simulink library "myLibrary"  (R2023b)
settings: Solver=VariableStepAuto  StartTime=0.0  StopTime=10.0  RelTol=1e-3
undefined symbols (not defined in the file): Cac_n1, ctrl1, Da, delta_slk, Discrete, dtha, ee_sli_rtmsupport, FA, gcbh, Ha, Ini, init_DCline, init_IPC, init_line, init_load, init_SG, init_shunt, init_TH, init_trafo, init_user, init_VSC, initMachineBlocks, Ka, Lf, Llkd_pu, Llkq1_pu, magnitude, NET, P, plots_step, q0, Rac_n1, Radd, Rkd_pu, Rkq1_pu, Rload_add, sim_config, sps_rtmsupport, spsSteamTurbineModel, T_DC_NET, T_global, T_IPC, T_load, T_NET, T_SG, T_shunt, T_STATCOM, T_TH, T_trafo, T_user, T_VSC, Ts, tstep, Udiff_a, V1
libraries: spsSeriesRLCBranchLib x120, eeGeneralControl x83, $bdroot x78, spsCurrentMeasurementLib x53, spsParallelRLCBranchLib x39, spsVoltageMeasurementLib x37, spsControlledVoltageSourceLib x30, simulink x29, spsFirstOrderFilterLib x18, spsMeasurementModel x13, spsThreePhaseVIMeasurementLib x5, dspsigops x4
(part 12 of 16)

== system myLibrary/SG_step/Governor-Turbine/Steam Turbine and Governor ==
  wref : Inport
  Pref : Inport  Port=2
  wm : Inport  Port=3
  d_theta : Inport  Port=4
  Model : Subsystem  AncestorBlock=spsSteamTurbineModel/Discrete  DialogController=POWERSYS.PowerSysDialog
      settings: LibrarySourceBlock=spsSteamTurbineModel/Discrete
  dw_5-2 : Outport  VectorParamsAs1DForOutWhenUnconnected=off
  Tr5-2 : Outport  Port=2  VectorParamsAs1DForOutWhenUnconnected=off
  gate : Outport  Port=3  VectorParamsAs1DForOutWhenUnconnected=off
  Pm : Outport  Port=4  VectorParamsAs1DForOutWhenUnconnected=off
  wires:
  wm/1 -> Model/4(wm)
  Model/4(gate) -> gate/1
  Model/3(dw_5-2) -> dw_5-2/1
  d_theta/1 -> Model/3(d_theta)
  Model/2(Tr5-2) -> Tr5-2/1
  Model/1(Pm) -> Pm/1
  wref/1 -> Model/2(wref)
  Pref/1 -> Model/1(Pref)

== system myLibrary/STATCOM/Control/Clarke Anti-Transformation ==
  V_alfa_diff : Inport
  V_beta_dfff : Inport  Port=2
  V_0_diff : Inport  Port=3
  Constant{,2,5,8} (4 alike) : Constant
  Constant1 : Constant  Value=0
  Constant3 : Constant  Value=-1/2
  Constant4 : Constant  Value=-sqrt(3)/2
  Constant6 : Constant  Value=-1/2
  Constant7 : Constant  Value=sqrt(3)/2
  Demux : Demux  Outputs=3
  Display : Display
  Math Function : Math  Operator=transpose  SignedPower=on
  Matrix Concatenate : Concatenate  NumInputs=3  Mode=Multidimensional array  ConcatenateDimension=2
  Mux{,1..3} (4 alike) : Mux  Inputs=3
  Product : Product  Multiplication=Matrix(*)
  Va_diff : Outport  VectorParamsAs1DForOutWhenUnconnected=off
  Vb_diff : Outport  Port=2  VectorParamsAs1DForOutWhenUnconnected=off
  Vc_diff : Outport  Port=3  VectorParamsAs1DForOutWhenUnconnected=off
  wires:
  V_0_diff/1 -> Mux/3  "0"
  V_beta_dfff/1 -> Mux/2  "Vbeta"
  V_alfa_diff/1 -> Mux/1  "Valfa"
  Math Function/1 -> Product/1, Display/1
  Mux/1 -> Product/2
  Demux/3 -> Vc_diff/1  "Vc"
  Demux/2 -> Vb_diff/1  "Vb"
  Demux/1 -> Va_diff/1  "Va"
  Product/1 -> Demux/1
  Mux1/1 -> Matrix Concatenate/1
  Mux3/1 -> Matrix Concatenate/3
  Mux2/1 -> Matrix Concatenate/2
  Matrix Concatenate/1 -> Math Function/1
  Constant8/1 -> Mux3/3
  Constant7/1 -> Mux3/2
  Constant6/1 -> Mux3/1
  Constant5/1 -> Mux2/3
  Constant4/1 -> Mux2/2
  Constant3/1 -> Mux2/1
  Constant2/1 -> Mux1/3
  Constant1/1 -> Mux1/2
  Constant/1 -> Mux1/1

== system myLibrary/STATCOM/Control/Conditional unit delay ==
  In1 : Inport
  Constant4 : Constant  Value=T_VSC.tau_cmd
  Switch : Switch  Criteria=u2 > Threshold  SaturateOnIntegerOverflow=off  InputSameDT=off
  Unit Delay2 : UnitDelay  InitialCondition=initVSC.vdiffq  SampleTime=T_VSC.tau_cmd  HasFrameUpgradeWarning=on
  Out1 : Outport
  wires:
  Switch/1 -> Out1/1
  Unit Delay2/1 -> Switch/1
  In1/1 -> Switch/3, Unit Delay2/1
  Constant4/1 -> Switch/2

== system myLibrary/STATCOM/Control/Conditional zoh ==
  In1 : Inport
  Constant4 : Constant  Value=T_VSC.tau_zoh
  Switch : Switch  Criteria=u2 > Threshold  SaturateOnIntegerOverflow=off  InputSameDT=off
  Zero-Order Hold9 : ZeroOrderHold  SampleTime=T_VSC.tau_zoh
  Out1 : Outport
  wires:
  Switch/1 -> Out1/1
  Constant4/1 -> Switch/2
  Zero-Order Hold9/1 -> Switch/1
  In1/1 -> Switch/3, Zero-Order Hold9/1

== system myLibrary/STATCOM/Control/Current Control ==
  Iq* : Inport
  Iq : Inport  Port=2
  Id* : Inport  Port=3
  Id : Inport  Port=4
  uq : Inport  Port=5
  ud : Inport  Port=6
  Constant : Constant  Value=T_VSC.wb
  Id1 : InportShadow  Port=4
  Integrator : Integrator  InitialCondition=initVSC.PI_idiffq
  Integrator1 : Integrator  InitialCondition=initVSC.PI_idiffd
  Iq1 : InportShadow  Port=2
  Ki : Gain  Gain=T_VSC.ki_s
  Ki1 : Gain  Gain=T_VSC.ki_s
  Kp : Gain  Gain=T_VSC.kp_s
  Kp1 : Gain  Gain=T_VSC.kp_s
  Lc : Gain  Gain=T_VSC.Lc
  Product : Product
  Product1 : Product
  Scope : Scope  NumInputPorts=2
  Sum : Sum  Inputs=|+-
  Sum1 : Sum  Inputs=|+-
  Sum2 : Sum  Inputs=+++
  Sum3 : Sum  Inputs=-++
  Sum4 : Sum
  Sum5 : Sum
  V_q_s : Outport  VectorParamsAs1DForOutWhenUnconnected=off
  V_d_s : Outport  Port=2  VectorParamsAs1DForOutWhenUnconnected=off
  wires:
  Id*/1 -> Sum1/1, Scope/1
  Integrator/1 -> Sum4/1
  Id1/1 -> Product1/2
  Iq1/1 -> Product/1
  Product1/1 -> Sum2/2
  Product/1 -> Sum3/1
  Sum3/1 -> V_d_s/1
  uq/1 -> Sum2/3
  Sum4/1 -> Sum2/1
  ud/1 -> Sum3/3
  Constant/1 -> Lc/1
  Iq*/1 -> Sum/1
  Iq/1 -> Sum/2
  Id/1 -> Sum1/2, Scope/2
  Lc/1 -> Product1/1, Product/2
  Sum/1 -> Ki/1, Kp/1
  Ki/1 -> Integrator/1
  Kp/1 -> Sum4/2
  Sum1/1 -> Kp1/1, Ki1/1  "Error"
  Ki1/1 -> Integrator1/1
  Integrator1/1 -> Sum5/1
  Kp1/1 -> Sum5/2
  Sum5/1 -> Sum3/2
  Sum2/1 -> V_q_s/1

== system myLibrary/STATCOM/Control/DC voltage control ==
  Vdc : Inport
  Constant : Constant
  Integrator : Integrator  InitialCondition=-initVSC.idiffq
  Ki : Gain  Gain=T_VSC.kiVdc
  Kp : Gain  Gain=T_VSC.kpVdc
  Kp1 : Gain  Gain=-1
  Scope : Scope  NumInputPorts=2
  Scope1 : Scope
  Sum1 : Sum  Inputs=|+-
  Sum4 : Sum
  iq : Outport
  wires:
  Constant/1 -> Scope/1, Sum1/1
  Sum1/1 -> Kp/1, Ki/1
  Ki/1 -> Integrator/1
  Sum4/1 -> Kp1/1
  Vdc/1 -> Scope/2, Sum1/2
  Kp1/1 -> Scope1/1, iq/1
  Integrator/1 -> Sum4/1
  Kp/1 -> Sum4/2

== system myLibrary/STATCOM/Control/Is ==
  Ias : Inport
  Ibs : Inport  Port=2
  Ics : Inport  Port=3
  Angle : Inport  Port=4
  Demux1 : Demux  Outputs=3
  Matriu T : Subsystem
  Mux : Mux  Inputs=3
  Product : Product  Multiplication=Matrix(*)
  Terminator : Terminator
  I_q_s : Outport  VectorParamsAs1DForOutWhenUnconnected=off
  I_d_s : Outport  Port=2  VectorParamsAs1DForOutWhenUnconnected=off
  wires:
  Ics/1 -> Mux/3
  Ibs/1 -> Mux/2
  Ias/1 -> Mux/1
  Mux/1 -> Product/2
  Angle/1 -> Matriu T/1(u)
  Demux1/3 -> Terminator/1
  Demux1/2 -> I_d_s/1
  Demux1/1 -> I_q_s/1
  Matriu T/1(Out1) -> Product/1
  Product/1 -> Demux1/1

== system myLibrary/STATCOM/Control/Is1 ==
  Ias : Inport
  Ibs : Inport  Port=2
  Ics : Inport  Port=3
  Angle : Inport  Port=4
  Demux1 : Demux  Outputs=3
  Matriu T : Subsystem
  Mux : Mux  Inputs=3
  Product : Product  Multiplication=Matrix(*)
  I_q_s : Outport  VectorParamsAs1DForOutWhenUnconnected=off
  I_d_s : Outport  Port=2  VectorParamsAs1DForOutWhenUnconnected=off
  I_0_s : Outport  Port=3  VectorParamsAs1DForOutWhenUnconnected=off
  wires:
  Product/1 -> Demux1/1
  Matriu T/1(Out1) -> Product/1
  Demux1/1 -> I_q_s/1
  Demux1/2 -> I_d_s/1
  Demux1/3 -> I_0_s/1
  Angle/1 -> Matriu T/1(u)
  Mux/1 -> Product/2
  Ias/1 -> Mux/1
  Ibs/1 -> Mux/2
  Ics/1 -> Mux/3

== system myLibrary/STATCOM/Control/Is3 ==
  Ias : Inport
  Ibs : Inport  Port=2
  Ics : Inport  Port=3
  Angle : Inport  Port=4
  Demux1 : Demux  Outputs=3
  Matriu T : Subsystem
  Mux : Mux  Inputs=3
  Product : Product  Multiplication=Matrix(*)
  I_q_s : Outport  VectorParamsAs1DForOutWhenUnconnected=off
  I_d_s : Outport  Port=2  VectorParamsAs1DForOutWhenUnconnected=off
  I_0_s : Outport  Port=3  VectorParamsAs1DForOutWhenUnconnected=off
  wires:
  Ics/1 -> Mux/3
  Ibs/1 -> Mux/2
  Ias/1 -> Mux/1
  Mux/1 -> Product/2
  Angle/1 -> Matriu T/1(u)
  Demux1/3 -> I_0_s/1
  Demux1/2 -> I_d_s/1
  Demux1/1 -> I_q_s/1
  Matriu T/1(Out1) -> Product/1
  Product/1 -> Demux1/1

== system myLibrary/STATCOM/Control/Is4 ==
  Ias : Inport
  Ibs : Inport  Port=2
  Ics : Inport  Port=3
  Angle : Inport  Port=4
  Demux1 : Demux  Outputs=3
  Matriu T : Subsystem
  Mux : Mux  Inputs=3
  Product : Product  Multiplication=Matrix(*)
  I_q_s : Outport  VectorParamsAs1DForOutWhenUnconnected=off
  I_d_s : Outport  Port=2  VectorParamsAs1DForOutWhenUnconnected=off
  I_0_s : Outport  Port=3  VectorParamsAs1DForOutWhenUnconnected=off
  wires:
  Product/1 -> Demux1/1
  Matriu T/1(Out1) -> Product/1
  Demux1/1 -> I_q_s/1
  Demux1/2 -> I_d_s/1
  Demux1/3 -> I_0_s/1
  Angle/1 -> Matriu T/1(u)
  Mux/1 -> Product/2
  Ias/1 -> Mux/1
  Ibs/1 -> Mux/2
  Ics/1 -> Mux/3

== system myLibrary/STATCOM/Control/Is5 ==
  Ias : Inport
  Ibs : Inport  Port=2
  Ics : Inport  Port=3
  Angle : Inport  Port=4
  Demux1 : Demux  Outputs=3
  Matriu T : Subsystem
  Mux : Mux  Inputs=3
  Product : Product  Multiplication=Matrix(*)
  I_q_s : Outport  VectorParamsAs1DForOutWhenUnconnected=off
  I_d_s : Outport  Port=2  VectorParamsAs1DForOutWhenUnconnected=off
  I_0_s : Outport  Port=3  VectorParamsAs1DForOutWhenUnconnected=off
  wires:
  Ics/1 -> Mux/3
  Ibs/1 -> Mux/2
  Ias/1 -> Mux/1
  Mux/1 -> Product/2
  Angle/1 -> Matriu T/1(u)
  Demux1/3 -> I_0_s/1
  Demux1/2 -> I_d_s/1
  Demux1/1 -> I_q_s/1
  Matriu T/1(Out1) -> Product/1
  Product/1 -> Demux1/1

== system myLibrary/STATCOM/Control/Is7 ==
  Ias : Inport
  Ibs : Inport  Port=2
  Ics : Inport  Port=3
  Angle : Inport  Port=4
  Demux1 : Demux  Outputs=3
  Matriu T : Subsystem
  Mux : Mux  Inputs=3
  Product : Product  Multiplication=Matrix(*)
  I_q_s : Outport  VectorParamsAs1DForOutWhenUnconnected=off
  I_d_s : Outport  Port=2  VectorParamsAs1DForOutWhenUnconnected=off
  I_0_s : Outport  Port=3  VectorParamsAs1DForOutWhenUnconnected=off
  wires:
  Product/1 -> Demux1/1
  Matriu T/1(Out1) -> Product/1
  Demux1/1 -> I_q_s/1
  Demux1/2 -> I_d_s/1
  Demux1/3 -> I_0_s/1
  Angle/1 -> Matriu T/1(u)
  Mux/1 -> Product/2
  Ias/1 -> Mux/1
  Ibs/1 -> Mux/2
  Ics/1 -> Mux/3

== system myLibrary/STATCOM/Control/PLL ==
  note: PLL
  U : Inport
  Ud : Inport  Port=2
  Constant : Constant  Value=0
  Constant1 : Constant
  Demux : Demux  Outputs=3
  Integrator : Integrator  InitialCondition=initVSC.thetaPLL_init
  Integrator1 : Integrator
  Ki : Gain  Gain=T_VSC.ki_pll
  Kp : Gain  Gain=T_VSC.kp_pll
  Scope1 : Scope
  Scope4 : Scope  NumInputPorts=2
  Sum : Sum  Inputs=|+-
  Sum1 : Sum  Inputs=|++
  Sum2 : Sum  Inputs=|++
  Terminator : Terminator
  Tpark : Subsystem
  wb : Gain  Gain=T_VSC.wb
  Angle : Outport
  Vzq : Outport  Port=2
  Vzd : Outport  Port=3
  w : Outport  Port=4
  wires:
  Ud/1 -> Sum/2, Scope4/2
  Tpark/1(Vq) -> Vzq/1
  U/1 -> Demux/1
  Demux/2 -> Tpark/2(Vb)
  Demux/3 -> Tpark/3(Vc)
  Demux/1 -> Tpark/1(Va)
  Constant/1 -> Sum/1, Scope4/1
  Sum/1 -> Ki/1, Kp/1
  Ki/1 -> Integrator1/1
  Kp/1 -> Sum1/1
  Integrator1/1 -> Sum1/2
  Integrator/1 -> Tpark/4(u), Angle/1
  Tpark/3(0) -> Terminator/1
  Sum1/1 -> Sum2/1
  Constant1/1 -> Sum2/2
  Tpark/2(Vd) -> Vzd/1
  Sum2/1 -> wb/1, Scope1/1
  wb/1 -> w/1, Integrator/1

== system myLibrary/STATCOM/Control/POD ==
  Uq : Inport
  Ud : Inport  Port=2
  iq : Inport  Port=3
  id : Inport  Port=4
  Gain : Gain  Gain=3/2
  LPF : TransferFcn  Denominator=[T_VSC.TLPF 1]
  LeadLag : TransferFcn  Numerator=[T_VSC.T1 1]  Denominator=[T_VSC.T2 1]
  Product : Product
  Product1 : Product
  Sum : Sum
  WashOut : TransferFcn  Numerator=[T_VSC.T 0]  Denominator=[T_VSC.T 1]
  Id_ref : Outport
  wires:
  Uq/1 -> Product/1
  iq/1 -> Product/2
  Ud/1 -> Product1/1
  id/1 -> Product1/2
  Product/1 -> Sum/1
  Product1/1 -> Sum/2
  Sum/1 -> Gain/1
  WashOut/1 -> LeadLag/1
  LeadLag/1 -> Id_ref/1
  LPF/1 -> WashOut/1
  Gain/1 -> LPF/1

== system myLibrary/STATCOM/Control/Rotació ==
  V_q_diff : Inport
  V_d_diff : Inport  Port=2
  V_0_diff : Inport  Port=3
  Angle : Inport  Port=4
  Constant{2,5..7} (4 alike) : Constant  Value=0
  Constant8 : Constant
  Demux : Demux  Outputs=3
  Display : Display
  Gain1 : Gain  Gain=-1
  Matrix Concatenate : Concatenate  NumInputs=3  Mode=Multidimensional array  ConcatenateDimension=2
  Mux{,1..3} (4 alike) : Mux  Inputs=3
  Product : Product  Multiplication=Matrix(*)
  Trigonometric Function : Trigonometry  Operator=cos
  Trigonometric Function1 : Trigonometry
  Trigonometric Function2 : Trigonometry
  Trigonometric Function3 : Trigonometry  Operator=cos
  V_alfa_diff : Outport  VectorParamsAs1DForOutWhenUnconnected=off
  V_beta_diff : Outport  Port=2  VectorParamsAs1DForOutWhenUnconnected=off
  V_0 : Outport  Port=3  VectorParamsAs1DForOutWhenUnconnected=off
  wires:
  Angle/1 -> Trigonometric Function1/1, Trigonometric Function2/1, Trigonometric Function3/1, Trigonometric Function/1
  Trigonometric Function2/1 -> Mux2/1
  Gain1/1 -> Mux1/2
  Trigonometric Function/1 -> Mux1/1
  V_0_diff/1 -> Mux/3
  V_d_diff/1 -> Mux/2
  V_q_diff/1 -> Mux/1
  Matrix Concatenate/1 -> Product/1, Display/1
  Mux/1 -> Product/2
  Demux/3 -> V_0/1
  Demux/2 -> V_beta_diff/1
  Demux/1 -> V_alfa_diff/1
  Product/1 -> Demux/1
  Mux1/1 -> Matrix Concatenate/1
  Mux3/1 -> Matrix Concatenate/3
  Mux2/1 -> Matrix Concatenate/2
  Constant8/1 -> Mux3/3
  Constant7/1 -> Mux3/2
  Constant6/1 -> Mux3/1
  Constant5/1 -> Mux2/3
  Trigonometric Function3/1 -> Mux2/2
  Constant2/1 -> Mux1/3
  Trigonometric Function1/1 -> Gain1/1

== system myLibrary/STATCOM/Control/Subsystem ==
  Uq : Inport
  Ud : Inport  Port=2
  iq : Inport  Port=3
  id : Inport  Port=4
  Gain2 : Gain  Gain=3/2
  Product : Product
  Product1 : Product
  Sum8 : Sum
  Pac : Outport
  wires:
  Uq/1 -> Product/1
  Product/1 -> Sum8/1
  iq/1 -> Product/2
  id/1 -> Product1/2
  Gain2/1 -> Pac/1
  Ud/1 -> Product1/1
  Product1/1 -> Sum8/2
  Sum8/1 -> Gain2/1

== system myLibrary/WT/Control/Clarke Anti-Transformation ==
  V_alfa_diff : Inport
  V_beta_dfff : Inport  Port=2
  V_0_diff : Inport  Port=3
  Constant{,2,5,8} (4 alike) : Constant
  Constant1 : Constant  Value=0
  Constant3 : Constant  Value=-1/2
  Constant4 : Constant  Value=-sqrt(3)/2
  Constant6 : Constant  Value=-1/2
  Constant7 : Constant  Value=sqrt(3)/2
  Demux : Demux  Outputs=3
  Display : Display
  Math Function : Math  Operator=transpose  SignedPower=on
  Matrix Concatenate : Concatenate  NumInputs=3  Mode=Multidimensional array  ConcatenateDimension=2
  Mux{,1..3} (4 alike) : Mux  Inputs=3
  Product : Product  Multiplication=Matrix(*)
  Va_diff : Outport  VectorParamsAs1DForOutWhenUnconnected=off
  Vb_diff : Outport  Port=2  VectorParamsAs1DForOutWhenUnconnected=off
  Vc_diff : Outport  Port=3  VectorParamsAs1DForOutWhenUnconnected=off
  wires:
  V_0_diff/1 -> Mux/3  "0"
  V_beta_dfff/1 -> Mux/2  "Vbeta"
  V_alfa_diff/1 -> Mux/1  "Valfa"
  Math Function/1 -> Product/1, Display/1
  Mux/1 -> Product/2
  Demux/3 -> Vc_diff/1  "Vc"
  Demux/2 -> Vb_diff/1  "Vb"
  Demux/1 -> Va_diff/1  "Va"
  Product/1 -> Demux/1
  Mux1/1 -> Matrix Concatenate/1
  Mux3/1 -> Matrix Concatenate/3
  Mux2/1 -> Matrix Concatenate/2
  Matrix Concatenate/1 -> Math Function/1
  Constant8/1 -> Mux3/3
  Constant7/1 -> Mux3/2
  Constant6/1 -> Mux3/1
  Constant5/1 -> Mux2/3
  Constant4/1 -> Mux2/2
  Constant3/1 -> Mux2/1
  Constant2/1 -> Mux1/3
  Constant1/1 -> Mux1/2
  Constant/1 -> Mux1/1

== system myLibrary/WT/Control/Current Control ==
  Iq* : Inport
  Iq : Inport  Port=2
  Id* : Inport  Port=3
  Id : Inport  Port=4
  uq : Inport  Port=5
  ud : Inport  Port=6
  igq : Inport  Port=7
  igd : Inport  Port=8
  Constant : Constant  Value=T_VSC.wb
  Gain1 : Gain  Gain=T_VSC.cc_damp
  Gain2 : Gain  Gain=T_VSC.cc_damp
  Id1 : InportShadow  Port=4
  Id2 : InportShadow  Port=4
  Integrator : Integrator  InitialCondition=initVSC.PI_idiffq
  Integrator1 : Integrator  InitialCondition=initVSC.PI_idiffd
  Iq1 : InportShadow  Port=2
  Iq2 : InportShadow  Port=2
  Ki : Gain  Gain=T_VSC.ki_s
  Ki1 : Gain  Gain=T_VSC.ki_s
  Kp : Gain  Gain=T_VSC.kp_s
  Kp1 : Gain  Gain=T_VSC.kp_s
  Lc : Gain  Gain=T_VSC.Lc
  Lc1 : Gain  Gain=T_VSC.Rc*T_VSC.Lc*T_VSC.wb
  Lc2 : Gain  Gain=T_VSC.Rc*T_VSC.Lc*T_VSC.wb
  Product : Product
  Product1 : Product
  Scope : Scope  NumInputPorts=2
  Scope{1..4} (4 alike) : Scope
  Sum{,1,8..9} (4 alike) : Sum  Inputs=|+-
  Sum2 : Sum  Inputs=+++++
  Sum3 : Sum  Inputs=+-+++
  Sum4 : Sum
  Sum5 : Sum
  V_q_s : Outport  VectorParamsAs1DForOutWhenUnconnected=off
  V_d_s : Outport  Port=2  VectorParamsAs1DForOutWhenUnconnected=off
  wires:
  Id*/1 -> Sum1/1, Scope/1
  Integrator/1 -> Scope3/1, Sum4/1
  Id1/1 -> Lc1/1, Product1/2
  Iq1/1 -> Lc2/1, Product/1
  Sum3/1 -> Scope2/1, V_d_s/1
  Sum4/1 -> Sum2/2
  Constant/1 -> Lc/1
  Iq*/1 -> Sum/1
  Iq/1 -> Sum/2
  Id/1 -> Sum1/2, Scope/2
  Lc/1 -> Product1/1, Product/2
  Sum/1 -> Ki/1, Kp/1
  Ki/1 -> Integrator/1
  Kp/1 -> Sum4/2
  Sum1/1 -> Kp1/1, Ki1/1  "Error"
  Ki1/1 -> Integrator1/1
  Integrator1/1 -> Scope4/1, Sum5/1
  Kp1/1 -> Sum5/2
  Sum2/1 -> Scope1/1, V_q_s/1
  ud/1 -> Sum3/1
  igq/1 -> Sum8/1
  Gain1/1 -> Sum2/1
  Iq2/1 -> Sum8/2
  Sum8/1 -> Gain1/1
  igd/1 -> Sum9/1
  Id2/1 -> Sum9/2
  Sum9/1 -> Gain2/1
  uq/1 -> Sum2/5
  Gain2/1 -> Sum3/5
  Sum5/1 -> Sum3/4
  Lc2/1 -> Sum2/3
  Product1/1 -> Sum2/4
  Product/1 -> Sum3/2
  Lc1/1 -> Sum3/3

== system myLibrary/WT/Control/DC voltage control ==
  Vdc : Inport
  Constant : Constant  Value=2*sqrt(3/2)
  Integrator : Integrator  InitialCondition=-initVSC.idiffqc_p
  Ki : Gain  Gain=T_VSC.kiVdc
  Kp : Gain  Gain=T_VSC.kpVdc
  Kp1 : Gain  Gain=-1
  Scope : Scope  NumInputPorts=2
  Scope1 : Scope
  Scope2 : Scope
  Sum1 : Sum  Inputs=|+-
  Sum4 : Sum
  iq : Outport
  wires:
  Constant/1 -> Scope/1, Sum1/1
  Sum1/1 -> Kp/1, Ki/1
  Ki/1 -> Integrator/1
  Sum4/1 -> Kp1/1
  Vdc/1 -> Scope/2, Sum1/2
  Kp1/1 -> Scope1/1, iq/1
  Integrator/1 -> Scope2/1, Sum4/1
  Kp/1 -> Sum4/2

== system myLibrary/WT/Control/Is ==
  Ias : Inport
  Ibs : Inport  Port=2
  Ics : Inport  Port=3
  Angle : Inport  Port=4
  Demux1 : Demux  Outputs=3
  Matriu T : Subsystem
  Mux : Mux  Inputs=3
  Product : Product  Multiplication=Matrix(*)
  Terminator : Terminator
  I_q_s : Outport  VectorParamsAs1DForOutWhenUnconnected=off
  I_d_s : Outport  Port=2  VectorParamsAs1DForOutWhenUnconnected=off
  wires:
  Ics/1 -> Mux/3
  Ibs/1 -> Mux/2
  Ias/1 -> Mux/1
  Mux/1 -> Product/2
  Angle/1 -> Matriu T/1(u)
  Demux1/3 -> Terminator/1
  Demux1/2 -> I_d_s/1
  Demux1/1 -> I_q_s/1
  Matriu T/1(Out1) -> Product/1
  Product/1 -> Demux1/1

== system myLibrary/WT/Control/Is1 ==
  Ias : Inport
  Ibs : Inport  Port=2
  Ics : Inport  Port=3
  Angle : Inport  Port=4
  Demux1 : Demux  Outputs=3
  Matriu T : Subsystem
  Mux : Mux  Inputs=3
  Product : Product  Multiplication=Matrix(*)
  I_q_s : Outport  VectorParamsAs1DForOutWhenUnconnected=off
  I_d_s : Outport  Port=2  VectorParamsAs1DForOutWhenUnconnected=off
  I_0_s : Outport  Port=3  VectorParamsAs1DForOutWhenUnconnected=off
  wires:
  Product/1 -> Demux1/1
  Matriu T/1(Out1) -> Product/1
  Demux1/1 -> I_q_s/1
  Demux1/2 -> I_d_s/1
  Demux1/3 -> I_0_s/1
  Angle/1 -> Matriu T/1(u)
  Mux/1 -> Product/2
  Ias/1 -> Mux/1
  Ibs/1 -> Mux/2
  Ics/1 -> Mux/3

== system myLibrary/WT/Control/Is3 ==
  Ias : Inport
  Ibs : Inport  Port=2
  Ics : Inport  Port=3
  Angle : Inport  Port=4
  Demux1 : Demux  Outputs=3
  Matriu T : Subsystem
  Mux : Mux  Inputs=3
  Product : Product  Multiplication=Matrix(*)
  I_q_s : Outport  VectorParamsAs1DForOutWhenUnconnected=off
  I_d_s : Outport  Port=2  VectorParamsAs1DForOutWhenUnconnected=off
  I_0_s : Outport  Port=3  VectorParamsAs1DForOutWhenUnconnected=off
  wires:
  Ics/1 -> Mux/3
  Ibs/1 -> Mux/2
  Ias/1 -> Mux/1
  Mux/1 -> Product/2
  Angle/1 -> Matriu T/1(u)
  Demux1/3 -> I_0_s/1
  Demux1/2 -> I_d_s/1
  Demux1/1 -> I_q_s/1
  Matriu T/1(Out1) -> Product/1
  Product/1 -> Demux1/1

== system myLibrary/WT/Control/Is4 ==
  Ias : Inport
  Ibs : Inport  Port=2
  Ics : Inport  Port=3
  Angle : Inport  Port=4
  Demux1 : Demux  Outputs=3
  Matriu T : Subsystem
  Mux : Mux  Inputs=3
  Product : Product  Multiplication=Matrix(*)
  I_q_s : Outport  VectorParamsAs1DForOutWhenUnconnected=off
  I_d_s : Outport  Port=2  VectorParamsAs1DForOutWhenUnconnected=off
  I_0_s : Outport  Port=3  VectorParamsAs1DForOutWhenUnconnected=off
  wires:
  Product/1 -> Demux1/1
  Matriu T/1(Out1) -> Product/1
  Demux1/1 -> I_q_s/1
  Demux1/2 -> I_d_s/1
  Demux1/3 -> I_0_s/1
  Angle/1 -> Matriu T/1(u)
  Mux/1 -> Product/2
  Ias/1 -> Mux/1
  Ibs/1 -> Mux/2
  Ics/1 -> Mux/3

== system myLibrary/WT/Control/Is5 ==
  Ias : Inport
  Ibs : Inport  Port=2
  Ics : Inport  Port=3
  Angle : Inport  Port=4
  Demux1 : Demux  Outputs=3
  Matriu T : Subsystem
  Mux : Mux  Inputs=3
  Product : Product  Multiplication=Matrix(*)
  I_q_s : Outport  VectorParamsAs1DForOutWhenUnconnected=off
  I_d_s : Outport  Port=2  VectorParamsAs1DForOutWhenUnconnected=off
  I_0_s : Outport  Port=3  VectorParamsAs1DForOutWhenUnconnected=off
  wires:
  Ics/1 -> Mux/3
  Ibs/1 -> Mux/2
  Ias/1 -> Mux/1
  Mux/1 -> Product/2
  Angle/1 -> Matriu T/1(u)
  Demux1/3 -> I_0_s/1
  Demux1/2 -> I_d_s/1
  Demux1/1 -> I_q_s/1
  Matriu T/1(Out1) -> Product/1
  Product/1 -> Demux1/1

== system myLibrary/WT/Control/Is7 ==
  Ias : Inport
  Ibs : Inport  Port=2
  Ics : Inport  Port=3
  Angle : Inport  Port=4
  Demux1 : Demux  Outputs=3
  Matriu T : Subsystem
  Mux : Mux  Inputs=3
  Product : Product  Multiplication=Matrix(*)
  I_q_s : Outport  VectorParamsAs1DForOutWhenUnconnected=off
  I_d_s : Outport  Port=2  VectorParamsAs1DForOutWhenUnconnected=off
  I_0_s : Outport  Port=3  VectorParamsAs1DForOutWhenUnconnected=off
  wires:
  Product/1 -> Demux1/1
  Matriu T/1(Out1) -> Product/1
  Demux1/1 -> I_q_s/1
  Demux1/2 -> I_d_s/1
  Demux1/3 -> I_0_s/1
  Angle/1 -> Matriu T/1(u)
  Mux/1 -> Product/2
  Ias/1 -> Mux/1
  Ibs/1 -> Mux/2
  Ics/1 -> Mux/3

== system myLibrary/WT/Control/Is8 ==
  Ias : Inport
  Ibs : Inport  Port=2
  Ics : Inport  Port=3
  Angle : Inport  Port=4
  Demux1 : Demux  Outputs=3
  Matriu T : Subsystem
  Mux : Mux  Inputs=3
  Product : Product  Multiplication=Matrix(*)
  I_q_s : Outport  VectorParamsAs1DForOutWhenUnconnected=off
  I_d_s : Outport  Port=2  VectorParamsAs1DForOutWhenUnconnected=off
  I_0_s : Outport  Port=3  VectorParamsAs1DForOutWhenUnconnected=off
  wires:
  Ics/1 -> Mux/3
  Ibs/1 -> Mux/2
  Ias/1 -> Mux/1
  Mux/1 -> Product/2
  Angle/1 -> Matriu T/1(u)
  Demux1/3 -> I_0_s/1
  Demux1/2 -> I_d_s/1
  Demux1/1 -> I_q_s/1
  Matriu T/1(Out1) -> Product/1
  Product/1 -> Demux1/1

== system myLibrary/WT/Control/Low-Pass Filter (Discrete or Continuous)2 ==
  u : Inport
  1/T : Product  Inputs=/*
  Enable/disable time constant : Subsystem
  Initialization : Subsystem  Variant=on  VariantControlMode=label  LabelModeActiveChoice=Init_param
  Integrator (Discrete or Continuous) : eeGeneralControl/Integrator (Discrete or Continuous)  LabelModeActiveChoice=Discrete  ExternalReset=level  LimitType=Anti-windup  B=B  A=A  Ts=Ts
      settings: LibrarySourceBlock=|
      | ee_sl_lib/General Control/Low-Pass Filter
      | (Discrete or Continuous)/Integrator
      | (Discrete or Continuous)
  K : Gain  Gain=K
  Sum1 : Sum  Inputs=-+|
  y : Outport  VectorParamsAs1DForOutWhenUnconnected=off
  wires:
  Initialization/1(x0) -> Integrator (Discrete or Continuous)/3
  u/1 -> K/1
  Enable/disable time constant/2(reset) -> Integrator (Discrete or Continuous)/2
  Integrator (Discrete or Continuous)/1 -> y/1, Enable/disable time constant/1(x), Sum1/1
  Enable/disable time constant/1(max(T,Ts)) -> 1/T/1
  1/T/1 -> Integrator (Discrete or Continuous)/1
  Sum1/1 -> 1/T/2
  K/1 -> Sum1/2, Initialization/1(u)

== system myLibrary/WT/Control/Low-Pass Filter (Discrete or Continuous)3 ==
  u : Inport
  1/T : Product  Inputs=/*
  Enable/disable time constant : Subsystem
  Initialization : Subsystem  Variant=on  VariantControlMode=label  LabelModeActiveChoice=Init_param
  Integrator (Discrete or Continuous) : eeGeneralControl/Integrator (Discrete or Continuous)  LabelModeActiveChoice=Discrete  ExternalReset=level  LimitType=Anti-windup  B=B  A=A  Ts=Ts
      settings: LibrarySourceBlock=|
      | ee_sl_lib/General Control/Low-Pass Filter
      | (Discrete or Continuous)/Integrator
      | (Discrete or Continuous)
  K : Gain  Gain=K
  Sum1 : Sum  Inputs=-+|
  y : Outport  VectorParamsAs1DForOutWhenUnconnected=off
  wires:
  Initialization/1(x0) -> Integrator (Discrete or Continuous)/3
  u/1 -> K/1
  Enable/disable time constant/2(reset) -> Integrator (Discrete or Continuous)/2
  Integrator (Discrete or Continuous)/1 -> y/1, Enable/disable time constant/1(x), Sum1/1
  Enable/disable time constant/1(max(T,Ts)) -> 1/T/1
  1/T/1 -> Integrator (Discrete or Continuous)/1
  Sum1/1 -> 1/T/2
  K/1 -> Sum1/2, Initialization/1(u)

== system myLibrary/WT/Control/Low-Pass Filter (Discrete or Continuous)4 ==
  u : Inport
  1/T : Product  Inputs=/*
  Enable/disable time constant : Subsystem
  Initialization : Subsystem  Variant=on  VariantControlMode=label  LabelModeActiveChoice=Init_param
  Integrator (Discrete or Continuous) : eeGeneralControl/Integrator (Discrete or Continuous)  LabelModeActiveChoice=Discrete  ExternalReset=level  LimitType=Anti-windup  B=B  A=A  Ts=Ts
      settings: LibrarySourceBlock=|
      | eeGeneralControl/Low-Pass Filter
      | (Discrete or Continuous)/Integrator
      | (Discrete or Continuous)
  K : Gain  Gain=K
  Sum1 : Sum  Inputs=-+|
  y : Outport  VectorParamsAs1DForOutWhenUnconnected=off
  wires:
  Initialization/1(x0) -> Integrator (Discrete or Continuous)/3
  u/1 -> K/1
  Enable/disable time constant/2(reset) -> Integrator (Discrete or Continuous)/2
  Integrator (Discrete or Continuous)/1 -> y/1, Enable/disable time constant/1(x), Sum1/1
  Enable/disable time constant/1(max(T,Ts)) -> 1/T/1
  1/T/1 -> Integrator (Discrete or Continuous)/1
  Sum1/1 -> 1/T/2
  K/1 -> Sum1/2, Initialization/1(u)

== system myLibrary/WT/Control/Low-Pass Filter (Discrete or Continuous)5 ==
  u : Inport
  1/T : Product  Inputs=/*
  Enable/disable time constant : Subsystem
  Initialization : Subsystem  Variant=on  VariantControlMode=label  LabelModeActiveChoice=Init_param
  Integrator (Discrete or Continuous) : eeGeneralControl/Integrator (Discrete or Continuous)  LabelModeActiveChoice=Discrete  ExternalReset=level  LimitType=Anti-windup  B=B  A=A  Ts=Ts
      settings: LibrarySourceBlock=|
      | ee_sl_lib/General Control/Low-Pass Filter
      | (Discrete or Continuous)/Integrator
      | (Discrete or Continuous)
  K : Gain  Gain=K
  Sum1 : Sum  Inputs=-+|
  y : Outport  VectorParamsAs1DForOutWhenUnconnected=off
  wires:
  K/1 -> Initialization/1(u), Sum1/2
  Sum1/1 -> 1/T/2
  1/T/1 -> Integrator (Discrete or Continuous)/1
  Enable/disable time constant/1(max(T,Ts)) -> 1/T/1
  Integrator (Discrete or Continuous)/1 -> Sum1/1, Enable/disable time constant/1(x), y/1
  Enable/disable time constant/2(reset) -> Integrator (Discrete or Continuous)/2
  u/1 -> K/1
  Initialization/1(x0) -> Integrator (Discrete or Continuous)/3

== system myLibrary/WT/Control/Low-Pass Filter (Discrete or Continuous)6 ==
  u : Inport
  1/T : Product  Inputs=/*
  Enable/disable time constant : Subsystem
  Initialization : Subsystem  Variant=on  VariantControlMode=label  LabelModeActiveChoice=Init_param
  Integrator (Discrete or Continuous) : eeGeneralControl/Integrator (Discrete or Continuous)  LabelModeActiveChoice=Discrete  ExternalReset=level  LimitType=Anti-windup  B=B  A=A  Ts=Ts
      settings: LibrarySourceBlock=|
      | ee_sl_lib/General Control/Low-Pass Filter
      | (Discrete or Continuous)/Integrator
      | (Discrete or Continuous)
  K : Gain  Gain=K
  Sum1 : Sum  Inputs=-+|
  y : Outport  VectorParamsAs1DForOutWhenUnconnected=off
  wires:
  K/1 -> Initialization/1(u), Sum1/2
  Sum1/1 -> 1/T/2
  1/T/1 -> Integrator (Discrete or Continuous)/1
  Enable/disable time constant/1(max(T,Ts)) -> 1/T/1
  Integrator (Discrete or Continuous)/1 -> Sum1/1, Enable/disable time constant/1(x), y/1
  Enable/disable time constant/2(reset) -> Integrator (Discrete or Continuous)/2
  u/1 -> K/1
  Initialization/1(x0) -> Integrator (Discrete or Continuous)/3

== system myLibrary/WT/Control/Low-Pass Filter (Discrete or Continuous)7 ==
  u : Inport
  1/T : Product  Inputs=/*
  Enable/disable time constant : Subsystem
  Initialization : Subsystem  Variant=on  VariantControlMode=label  LabelModeActiveChoice=Init_param
  Integrator (Discrete or Continuous) : eeGeneralControl/Integrator (Discrete or Continuous)  LabelModeActiveChoice=Discrete  ExternalReset=level  LimitType=Anti-windup  B=B  A=A  Ts=Ts
      settings: LibrarySourceBlock=|
      | ee_sl_lib/General Control/Low-Pass Filter
      | (Discrete or Continuous)/Integrator
      | (Discrete or Continuous)
  K : Gain  Gain=K
  Sum1 : Sum  Inputs=-+|
  y : Outport  VectorParamsAs1DForOutWhenUnconnected=off
  wires:
  Initialization/1(x0) -> Integrator (Discrete or Continuous)/3
  u/1 -> K/1
  Enable/disable time constant/2(reset) -> Integrator (Discrete or Continuous)/2
  Integrator (Discrete or Continuous)/1 -> y/1, Enable/disable time constant/1(x), Sum1/1
  Enable/disable time constant/1(max(T,Ts)) -> 1/T/1
  1/T/1 -> Integrator (Discrete or Continuous)/1
  Sum1/1 -> 1/T/2
  K/1 -> Sum1/2, Initialization/1(u)

== system myLibrary/WT/Control/Low-Pass Filter (Discrete or Continuous)8 ==
  u : Inport
  1/T : Product  Inputs=/*
  Enable/disable time constant : Subsystem
  Initialization : Subsystem  Variant=on  VariantControlMode=label  LabelModeActiveChoice=Init_param
  Integrator (Discrete or Continuous) : eeGeneralControl/Integrator (Discrete or Continuous)  LabelModeActiveChoice=Discrete  ExternalReset=level  LimitType=Anti-windup  B=B  A=A  Ts=Ts
      settings: LibrarySourceBlock=|
      | ee_sl_lib/General Control/Low-Pass Filter
      | (Discrete or Continuous)/Integrator
      | (Discrete or Continuous)
  K : Gain  Gain=K
  Sum1 : Sum  Inputs=-+|
  y : Outport  VectorParamsAs1DForOutWhenUnconnected=off
  wires:
  Initialization/1(x0) -> Integrator (Discrete or Continuous)/3
  u/1 -> K/1
  Enable/disable time constant/2(reset) -> Integrator (Discrete or Continuous)/2
  Integrator (Discrete or Continuous)/1 -> y/1, Enable/disable time constant/1(x), Sum1/1
  Enable/disable time constant/1(max(T,Ts)) -> 1/T/1
  1/T/1 -> Integrator (Discrete or Continuous)/1
  Sum1/1 -> 1/T/2
  K/1 -> Sum1/2, Initialization/1(u)

== system myLibrary/WT/Control/Low-Pass Filter (Discrete or Continuous)9 ==
  u : Inport
  1/T : Product  Inputs=/*
  Enable/disable time constant : Subsystem
  Initialization : Subsystem  Variant=on  VariantControlMode=label  LabelModeActiveChoice=Init_param
  Integrator (Discrete or Continuous) : eeGeneralControl/Integrator (Discrete or Continuous)  LabelModeActiveChoice=Discrete  ExternalReset=level  LimitType=Anti-windup  B=B  A=A  Ts=Ts
      settings: LibrarySourceBlock=|
      | ee_sl_lib/General Control/Low-Pass Filter
      | (Discrete or Continuous)/Integrator
      | (Discrete or Continuous)
  K : Gain  Gain=K
  Sum1 : Sum  Inputs=-+|
  y : Outport  VectorParamsAs1DForOutWhenUnconnected=off
  wires:
  K/1 -> Initialization/1(u), Sum1/2
  Sum1/1 -> 1/T/2
  1/T/1 -> Integrator (Discrete or Continuous)/1
  Enable/disable time constant/1(max(T,Ts)) -> 1/T/1
  Integrator (Discrete or Continuous)/1 -> Sum1/1, Enable/disable time constant/1(x), y/1
  Enable/disable time constant/2(reset) -> Integrator (Discrete or Continuous)/2
  u/1 -> K/1
  Initialization/1(x0) -> Integrator (Discrete or Continuous)/3

== system myLibrary/WT/Control/PLL ==
  note: PLL
  U : Inport
  Constant : Constant  Value=0
  Constant1 : Constant
  Demux : Demux  Outputs=3
  Integrator : Integrator  InitialCondition=initVSC.thetaPLL_init_filts
  Integrator1 : Integrator
  Ki : Gain  Gain=T_VSC.ki_pll
  Kp : Gain  Gain=T_VSC.kp_pll
  Low-Pass Filter (Discrete or Continuous)1 : Subsystem  LoadFcn=ee_sli_rtmsupport( 'loadfcn', gcbh );  mask(Low-Pass Filter (Discrete or Continuous)){K=1, T=0, B=inf, A=-inf, init_option=Specify as parameter, x0=initVSC.udc_p, Ts=-1}
      mask prompts: K "physmod:ee:library:comments:control:eeGeneralControl:Gain_MP"; T "physmod:ee:library:comments:control:eeGeneralControl:TimeConstant_MP"; B "physmod:ee:library:comments:control:eeGeneralControl:UpperSaturationLimit_MP"; A "physmod:ee:library:comments:control:eeGeneralControl:LowerSaturationLimit_MP"; init_option "physmod:ee:library:comments:control:eeGeneralControl:Initialization_MP"; x0 "physmod:ee:library:comments:control:eeGeneralControl:InitialState_MP"; Ts "physmod:ee:library:comments:control:eeGeneralControl:SampleTime1ForInherited_MP"
      mask help: physmod:ee:library:comments:control:eeGeneralControl:LowPassFilterDiscreteOrContinuous_MD
      mask init:
      | timeDomain = ee.mask.initializeLowPassFilter(T,B,A,Ts);
      | 
      | ee.mask.callbackPopupInitialization(gcb);
      settings: CopyFcn=ee_sli_rtmsupport( 'copyfcn', gcbh );  DeleteFcn=ee_sli_rtmsupport( 'deletefcn', gcbh );  ModelCloseFcn=ee_sli_rtmsupport( 'modelclosefcn', gcbh );  PostSaveFcn=ee_sli_rtmsupport( 'postsavefcn', gcbh );  PreCopyFcn=ee_sli_rtmsupport( 'precopyfcn', gcbh );  OpenFcn=ee_sli_rtmsupport( 'openfcn', gcbh );  CloseFcn=ee_sli_rtmsupport( 'closefcn', gcbh );  PreDeleteFcn=ee_sli_rtmsupport( 'predeletefcn', gcbh );
      settings: LibrarySourceBlock=|
      | eeGeneralControl/Low-Pass Filter
      | (Discrete or Continuous)
      mask Help: web(nesl_help(gcbh))
      mask TypeOptions init_option: physmod:ee:library:comments:control:eeGeneralControl:InheritedFromBlockInput_PV | physmod:ee:library:comments:control:eeGeneralControl:SpecifyAsParameter_PV
      mask Callback init_option: ee.mask.callbackPopupInitialization(gcb);
      mask TypeOptions Ts:
      | Integrator
      | (Discrete or Continuous)/Ts
      mask DialogControl ParameterGroupVar Prompt: physmod:ee:library:comments:control:eeGeneralControl:tab_Parameters
      mask DialogControl K Prompt: Gain
      mask DialogControl T Prompt: Time constant
      mask DialogControl B Prompt: Upper saturation limit
      mask DialogControl A Prompt: Lower saturation limit
      mask DialogControl init_option Prompt: Initialization
      mask DialogControl x0 Prompt: Initial state
      mask DialogControl Ts Prompt: Sample time (-1 for inherited)
      mask Display: ee.mask.drawLowPassFilter;
  Sum : Sum  Inputs=|+-
  Sum1 : Sum  Inputs=|++
  Sum2 : Sum  Inputs=|++
  Terminator : Terminator
  Tpark : Subsystem
  wb : Gain  Gain=T_VSC.wb
  Angle : Outport
  Vzq : Outport  Port=2
  Vzd : Outport  Port=3
  w : Outport  Port=4
  wires:
  Tpark/1(Vq) -> Vzq/1
  U/1 -> Demux/1
  Demux/2 -> Tpark/2(Vb)
  Demux/3 -> Tpark/3(Vc)
  Demux/1 -> Tpark/1(Va)
  Constant/1 -> Sum/1
  Sum/1 -> Ki/1, Kp/1
  Ki/1 -> Integrator1/1
  Kp/1 -> Sum1/1
  Integrator1/1 -> Sum1/2
  Integrator/1 -> Tpark/4(u), Angle/1
  Tpark/3(0) -> Terminator/1
  Sum1/1 -> Sum2/1
  Constant1/1 -> Sum2/2
  Tpark/2(Vd) -> Low-Pass Filter (Discrete or Continuous)1/1(u), Vzd/1
  Sum2/1 -> wb/1
  wb/1 -> w/1, Integrator/1
  Low-Pass Filter (Discrete or Continuous)1/1(y) -> Sum/2

== system myLibrary/WT/Control/Q control ==
  Q : Inport
  Integrator : Integrator  InitialCondition=initVSC.idiffdc_p
  Ki : Gain  Gain=T_VSC.ki_Q
  Kp : Gain  Gain=T_VSC.kp_Q
  Kp1 : Gain
  Scope : Scope
  Scope1 : Scope
  Sum4 : Sum
  id : Outport
  wires:
  Kp/1 -> Sum4/2
  Integrator/1 -> Scope/1, Sum4/1
  Kp1/1 -> id/1, Scope1/1
  Sum4/1 -> Kp1/1
  Ki/1 -> Integrator/1
  Q/1 -> Kp/1, Ki/1

== system myLibrary/WT/Control/Rotació ==
  V_q_diff : Inport
  V_d_diff : Inport  Port=2
  V_0_diff : Inport  Port=3
  Angle : Inport  Port=4
  Constant{2,5..7} (4 alike) : Constant  Value=0
  Constant8 : Constant
  Demux : Demux  Outputs=3
  Display : Display
  Gain1 : Gain  Gain=-1
  Matrix Concatenate : Concatenate  NumInputs=3  Mode=Multidimensional array  ConcatenateDimension=2
  Mux{,1..3} (4 alike) : Mux  Inputs=3
  Product : Product  Multiplication=Matrix(*)
  Trigonometric Function : Trigonometry  Operator=cos
  Trigonometric Function1 : Trigonometry
  Trigonometric Function2 : Trigonometry
  Trigonometric Function3 : Trigonometry  Operator=cos
  V_alfa_diff : Outport  VectorParamsAs1DForOutWhenUnconnected=off
  V_beta_diff : Outport  Port=2  VectorParamsAs1DForOutWhenUnconnected=off
  V_0 : Outport  Port=3  VectorParamsAs1DForOutWhenUnconnected=off
  wires:
  Angle/1 -> Trigonometric Function1/1, Trigonometric Function2/1, Trigonometric Function3/1, Trigonometric Function/1
  Trigonometric Function2/1 -> Mux2/1
  Gain1/1 -> Mux1/2
  Trigonometric Function/1 -> Mux1/1
  V_0_diff/1 -> Mux/3
  V_d_diff/1 -> Mux/2
  V_q_diff/1 -> Mux/1
  Matrix Concatenate/1 -> Product/1, Display/1
  Mux/1 -> Product/2
  Demux/3 -> V_0/1
  Demux/2 -> V_beta_diff/1
  Demux/1 -> V_alfa_diff/1
  Product/1 -> Demux/1
  Mux1/1 -> Matrix Concatenate/1
  Mux3/1 -> Matrix Concatenate/3
  Mux2/1 -> Matrix Concatenate/2
  Constant8/1 -> Mux3/3
  Constant7/1 -> Mux3/2
  Constant6/1 -> Mux3/1
  Constant5/1 -> Mux2/3
  Trigonometric Function3/1 -> Mux2/2
  Constant2/1 -> Mux1/3
  Trigonometric Function1/1 -> Gain1/1

== system myLibrary/WT/Control/Subsystem ==
  Uq : Inport
  Ud : Inport  Port=2
  iq : Inport  Port=3
  id : Inport  Port=4
  Product : Product
  Product1 : Product
  Sum8 : Sum
  Pac : Outport
  wires:
  Uq/1 -> Product/1
  Product/1 -> Sum8/1
  iq/1 -> Product/2
  id/1 -> Product1/2
  Sum8/1 -> Pac/1
  Ud/1 -> Product1/1
  Product1/1 -> Sum8/2

== system myLibrary/WT/Control/Subsystem1 ==
  Uq : Inport
  Ud : Inport  Port=2
  iq : Inport  Port=3
  id : Inport  Port=4
  Product : Product
  Product1 : Product
  Sum8 : Sum  Inputs=+-
  Qac : Outport
  wires:
  Product1/1 -> Sum8/2
  Ud/1 -> Product1/1
  Sum8/1 -> Qac/1
  Product/1 -> Sum8/1
  Uq/1 -> Product/1
  id/1 -> Product/2
  iq/1 -> Product1/2

== system myLibrary/WT/Electrical/Power7 ==
  Vabc : Inport  PortDimensions=3
  Iabc : Inport  Port=2  PortDimensions=3
  Demux : Demux  Outputs=3
      settings: DisplayOption=none
  Mux : Mux  Inputs=3
  Product1 : Product  InputSameDT=on  SaturateOnIntegerOverflow=on  OutDataTypeStr=Inherit: Same as first input
  Product3 : Product  InputSameDT=on  SaturateOnIntegerOverflow=on  OutDataTypeStr=Inherit: Same as first input
  Sum : Sum  Inputs=+-  InputSameDT=on  SaturateOnIntegerOverflow=on  OutDataTypeStr=Inherit: Same as first input
  Sum1 : Sum  Inputs=1  InputSameDT=on  SaturateOnIntegerOverflow=on  OutDataTypeStr=Inherit: Same as first input
  Sum4 : Sum  Inputs=1  InputSameDT=on  SaturateOnIntegerOverflow=on  OutDataTypeStr=Inherit: Same as first input
  Sum5 : Sum  Inputs=+-  InputSameDT=on  SaturateOnIntegerOverflow=on  OutDataTypeStr=Inherit: Same as first input
  Sum6 : Sum  Inputs=+-  InputSameDT=on  SaturateOnIntegerOverflow=on  OutDataTypeStr=Inherit: Same as first input
  pu->V : Gain  Gain=1/sqrt(3)  SaturateOnIntegerOverflow=on  OutDataTypeStr=Inherit: Same as input  ParamDataTypeStr=Inherit: Same as input
  P : Outport  VectorParamsAs1DForOutWhenUnconnected=off
  Q : Outport  Port=2  VectorParamsAs1DForOutWhenUnconnected=off
  wires:
  pu->V/1 -> Q/1
  Sum4/1 -> P/1
  Sum1/1 -> pu->V/1
  Product3/1 -> Sum1/1
  Product1/1 -> Sum4/1
  Vabc/1 -> Product1/1, Demux/1
  Iabc/1 -> Product1/2, Product3/2
  Demux/1 -> Sum/1, Sum6/2
  Demux/2 -> Sum/2, Sum5/1
  Demux/3 -> Sum5/2, Sum6/1
  Sum/1 -> Mux/3
  Sum5/1 -> Mux/1
  Sum6/1 -> Mux/2
  Mux/1 -> Product3/1

== system myLibrary/WT/Electrical/Voltage Measurement1 ==
  Model : spsMeasurementModel/Complex  SystemSampleTime=-1  VariantActivationTime=update diagram  AllowFlexibleInterface=on  Latency=0  AutoFrameSizeCalculation=off
      settings: LibrarySourceBlock=sps_lib/Sensors and Measurements/Voltage Measurement/Model
  VoltageMeasurement : PMComponent  PhysicalDomain=powersysdomain  LeftPortType=p1  RightPortType=p1  LConnTagsString=+  RConnTagsString=-  mask(InnerPowersysBlock){}
      mask Display: disp('SPS internal use\nDo not delete')
  do not delete this gain : Gain
  + : PMIOPort  Side=Left
  - : PMIOPort  Port=2  Side=Left
  v : Outport  InitialOutput=0  VectorParamsAs1DForOutWhenUnconnected=off
  wires:
  [T73_7485_8996354763478] -> Model/1
  do not delete this gain/1 -> v/1
  Model/1 -> do not delete this gain/1
  connections:
  +/RConn1 -- VoltageMeasurement/LConn1
  -/RConn1 -- VoltageMeasurement/RConn1

== system myLibrary/WT/Filter Ig/Second-Order Filter6 ==
  In : Inport  SampleTime=Ts
  Model : spsSecondOrderFilterModel/Continuous  SystemSampleTime=-1  VariantActivationTime=update diagram  AllowFlexibleInterface=on  Latency=0  AutoFrameSizeCalculation=off
  Out : Outport  SampleTime=Ts  InitialOutput=0  VectorParamsAs1DForOutWhenUnconnected=off
  wires:
  Model/1 -> Out/1
  In/1 -> Model/1

== system myLibrary/WT/Filter Is/Second-Order Filter3 ==
  In : Inport  SampleTime=Ts
  Model : spsSecondOrderFilterModel/Continuous  SystemSampleTime=-1  VariantActivationTime=update diagram  AllowFlexibleInterface=on  Latency=0  AutoFrameSizeCalculation=off
  Out : Outport  SampleTime=Ts  InitialOutput=0  VectorParamsAs1DForOutWhenUnconnected=off
  wires:
  In/1 -> Model/1
  Model/1 -> Out/1

== system myLibrary/WT/Filter Vdc/Second-Order Filter1 ==
  In : Inport  SampleTime=Ts
  Model : spsSecondOrderFilterModel/Continuous  SystemSampleTime=-1  VariantActivationTime=update diagram  AllowFlexibleInterface=on  Latency=0  AutoFrameSizeCalculation=off
  Out : Outport  SampleTime=Ts  InitialOutput=0  VectorParamsAs1DForOutWhenUnconnected=off
  wires:
  Model/1 -> Out/1
  In/1 -> Model/1

== system myLibrary/qd transform/qd0 Transformation/Matriu T ==
  u : Inport
  Constant : Constant  Value=(2/3)*[1/2 1/2 1/2]
  Fcn : Fcn  Expr=(2/3)*cos(u)
  Fcn1 : Fcn  Expr=(2/3)*cos(u-(2*pi)/3)
  Fcn2 : Fcn  Expr=(2/3)*cos(u+(2*pi)/3)
  Fcn3 : Fcn  Expr=(2/3)*sin(u)
  Fcn4 : Fcn  Expr=(2/3)*sin(u-(2*pi)/3)
  Fcn5 : Fcn  Expr=(2/3)*sin(u+(2*pi)/3)
  Math Function : Math  Operator=transpose  SignedPower=on
  Matrix Concatenate : Concatenate  NumInputs=3  Mode=Multidimensional array  ConcatenateDimension=2
  Mux : Mux  Inputs=3
  Mux1 : Mux  Inputs=3
  Out1 : Outport  VectorParamsAs1DForOutWhenUnconnected=off
  wires:
  u/1 -> Fcn/1, Fcn1/1, Fcn2/1, Fcn3/1, Fcn4/1, Fcn5/1
  Fcn3/1 -> Mux1/1
  Fcn4/1 -> Mux1/2
  Fcn5/1 -> Mux1/3
  Mux/1 -> Matrix Concatenate/1
  Constant/1 -> Matrix Concatenate/3
  Fcn/1 -> Mux/1
  Fcn1/1 -> Mux/2
  Fcn2/1 -> Mux/3
  Mux1/1 -> Matrix Concatenate/2
  Matrix Concatenate/1 -> Math Function/1
  Math Function/1 -> Out1/1

== system myLibrary/AC-GFOL_DC-GFOL/Control Pac2/Is/Matriu T ==
  u : Inport
  Constant : Constant  Value=(2/3)*[1/2 1/2 1/2]
  Fcn : Fcn  Expr=(2/3)*cos(u)
  Fcn1 : Fcn  Expr=(2/3)*cos(u-(2*pi)/3)
  Fcn2 : Fcn  Expr=(2/3)*cos(u+(2*pi)/3)
  Fcn3 : Fcn  Expr=(2/3)*sin(u)
  Fcn4 : Fcn  Expr=(2/3)*sin(u-(2*pi)/3)
  Fcn5 : Fcn  Expr=(2/3)*sin(u+(2*pi)/3)
  Math Function : Math  Operator=transpose  SignedPower=on
  Matrix Concatenate : Concatenate  NumInputs=3  Mode=Multidimensional array  ConcatenateDimension=2
  Mux : Mux  Inputs=3
  Mux1 : Mux  Inputs=3
  Out1 : Outport  VectorParamsAs1DForOutWhenUnconnected=off
  wires:
  u/1 -> Fcn/1, Fcn1/1, Fcn2/1, Fcn3/1, Fcn4/1, Fcn5/1
  Fcn3/1 -> Mux1/1
  Fcn4/1 -> Mux1/2
  Fcn5/1 -> Mux1/3
  Mux/1 -> Matrix Concatenate/1
  Constant/1 -> Matrix Concatenate/3
  Fcn/1 -> Mux/1
  Fcn1/1 -> Mux/2
  Fcn2/1 -> Mux/3
  Mux1/1 -> Matrix Concatenate/2
  Matrix Concatenate/1 -> Math Function/1
  Math Function/1 -> Out1/1

== system myLibrary/AC-GFOL_DC-GFOL/Control Pac2/Is2/Matriu T ==
  u : Inport
  Constant : Constant  Value=(2/3)*[1/2 1/2 1/2]
  Fcn : Fcn  Expr=(2/3)*cos(u)
  Fcn1 : Fcn  Expr=(2/3)*cos(u-(2*pi)/3)
  Fcn2 : Fcn  Expr=(2/3)*cos(u+(2*pi)/3)
  Fcn3 : Fcn  Expr=(2/3)*sin(u)
  Fcn4 : Fcn  Expr=(2/3)*sin(u-(2*pi)/3)
  Fcn5 : Fcn  Expr=(2/3)*sin(u+(2*pi)/3)
  Math Function : Math  Operator=transpose  SignedPower=on
  Matrix Concatenate : Concatenate  NumInputs=3  Mode=Multidimensional array  ConcatenateDimension=2
  Mux : Mux  Inputs=3
  Mux1 : Mux  Inputs=3
  Out1 : Outport  VectorParamsAs1DForOutWhenUnconnected=off
  wires:
  u/1 -> Fcn/1, Fcn1/1, Fcn2/1, Fcn3/1, Fcn4/1, Fcn5/1
  Fcn3/1 -> Mux1/1
  Fcn4/1 -> Mux1/2
  Fcn5/1 -> Mux1/3
  Mux/1 -> Matrix Concatenate/1
  Constant/1 -> Matrix Concatenate/3
  Fcn/1 -> Mux/1
  Fcn1/1 -> Mux/2
  Fcn2/1 -> Mux/3
  Mux1/1 -> Matrix Concatenate/2
  Matrix Concatenate/1 -> Math Function/1
  Math Function/1 -> Out1/1

== system myLibrary/AC-GFOL_DC-GFOL/Control Pac2/l_DC_alfa//beta/Clarke ==
  Isum : Inport
  Constant : Constant
  Constant1 : Constant  Value=-1/2
  Constant2 : Constant  Value=-1/2
  Constant3 : Constant  Value=0
  Constant4 : Constant  Value=-sqrt(3)/2
  Constant5 : Constant  Value=sqrt(3)/2
  Constant6 : Constant  Value=1/2
  Constant7 : Constant  Value=1/2
  Constant8 : Constant  Value=1/2
  Demux : Demux  Outputs=3
  Display : Display
  Gain : Gain  Gain=2/3
  Math Function : Math  Operator=transpose  SignedPower=on
  Matrix Concatenate : Concatenate  NumInputs=3  Mode=Multidimensional array  ConcatenateDimension=2
  Mux1 : Mux  Inputs=3
  Mux2 : Mux  Inputs=3
  Mux3 : Mux  Inputs=3
  Product : Product  Multiplication=Matrix(*)
  I_alfa : Outport  VectorParamsAs1DForOutWhenUnconnected=off
  I_beta : Outport  Port=2  VectorParamsAs1DForOutWhenUnconnected=off
  I_0 : Outport  Port=3  VectorParamsAs1DForOutWhenUnconnected=off
  wires:
  Constant/1 -> Mux1/1
  Constant1/1 -> Mux1/2
  Constant2/1 -> Mux1/3
  Constant3/1 -> Mux2/1
  Constant4/1 -> Mux2/2
  Constant5/1 -> Mux2/3
  Constant6/1 -> Mux3/1
  Constant7/1 -> Mux3/2
  Constant8/1 -> Mux3/3
  Math Function/1 -> Gain/1
  Matrix Concatenate/1 -> Math Function/1
  Mux2/1 -> Matrix Concatenate/2
  Mux3/1 -> Matrix Concatenate/3
  Mux1/1 -> Matrix Concatenate/1
  Product/1 -> Demux/1
  Demux/1 -> I_alfa/1
  Demux/2 -> I_beta/1
  Demux/3 -> I_0/1
  Gain/1 -> Display/1, Product/1
  Isum/1 -> Product/2

== system myLibrary/AC-GFOL_DC-GFOR/Control Pac2/Is/Matriu T ==
  u : Inport
  Constant : Constant  Value=(2/3)*[1/2 1/2 1/2]
  Fcn : Fcn  Expr=(2/3)*cos(u)
  Fcn1 : Fcn  Expr=(2/3)*cos(u-(2*pi)/3)
  Fcn2 : Fcn  Expr=(2/3)*cos(u+(2*pi)/3)
  Fcn3 : Fcn  Expr=(2/3)*sin(u)
  Fcn4 : Fcn  Expr=(2/3)*sin(u-(2*pi)/3)
  Fcn5 : Fcn  Expr=(2/3)*sin(u+(2*pi)/3)
  Math Function : Math  Operator=transpose  SignedPower=on
  Matrix Concatenate : Concatenate  NumInputs=3  Mode=Multidimensional array  ConcatenateDimension=2
  Mux : Mux  Inputs=3
  Mux1 : Mux  Inputs=3
  Out1 : Outport  VectorParamsAs1DForOutWhenUnconnected=off
  wires:
  u/1 -> Fcn/1, Fcn1/1, Fcn2/1, Fcn3/1, Fcn4/1, Fcn5/1
  Fcn3/1 -> Mux1/1
  Fcn4/1 -> Mux1/2
  Fcn5/1 -> Mux1/3
  Mux/1 -> Matrix Concatenate/1
  Constant/1 -> Matrix Concatenate/3
  Fcn/1 -> Mux/1
  Fcn1/1 -> Mux/2
  Fcn2/1 -> Mux/3
  Mux1/1 -> Matrix Concatenate/2
  Matrix Concatenate/1 -> Math Function/1
  Math Function/1 -> Out1/1

== system myLibrary/AC-GFOL_DC-GFOR/Control Pac2/Is2/Matriu T ==
  u : Inport
  Constant : Constant  Value=(2/3)*[1/2 1/2 1/2]
  Fcn : Fcn  Expr=(2/3)*cos(u)
  Fcn1 : Fcn  Expr=(2/3)*cos(u-(2*pi)/3)
  Fcn2 : Fcn  Expr=(2/3)*cos(u+(2*pi)/3)
  Fcn3 : Fcn  Expr=(2/3)*sin(u)
  Fcn4 : Fcn  Expr=(2/3)*sin(u-(2*pi)/3)
  Fcn5 : Fcn  Expr=(2/3)*sin(u+(2*pi)/3)
  Math Function : Math  Operator=transpose  SignedPower=on
  Matrix Concatenate : Concatenate  NumInputs=3  Mode=Multidimensional array  ConcatenateDimension=2
  Mux : Mux  Inputs=3
  Mux1 : Mux  Inputs=3
  Out1 : Outport  VectorParamsAs1DForOutWhenUnconnected=off
  wires:
  u/1 -> Fcn/1, Fcn1/1, Fcn2/1, Fcn3/1, Fcn4/1, Fcn5/1
  Fcn3/1 -> Mux1/1
  Fcn4/1 -> Mux1/2
  Fcn5/1 -> Mux1/3
  Mux/1 -> Matrix Concatenate/1
  Constant/1 -> Matrix Concatenate/3
  Fcn/1 -> Mux/1
  Fcn1/1 -> Mux/2
  Fcn2/1 -> Mux/3
  Mux1/1 -> Matrix Concatenate/2
  Matrix Concatenate/1 -> Math Function/1
  Math Function/1 -> Out1/1

== system myLibrary/AC-GFOL_DC-GFOR/Control Pac2/l_DC_alfa//beta/Clarke ==
  Isum : Inport
  Constant : Constant
  Constant1 : Constant  Value=-1/2
  Constant2 : Constant  Value=-1/2
  Constant3 : Constant  Value=0
  Constant4 : Constant  Value=-sqrt(3)/2
  Constant5 : Constant  Value=sqrt(3)/2
  Constant6 : Constant  Value=1/2
  Constant7 : Constant  Value=1/2
  Constant8 : Constant  Value=1/2
  Demux : Demux  Outputs=3
  Display : Display
  Gain : Gain  Gain=2/3
  Math Function : Math  Operator=transpose  SignedPower=on
  Matrix Concatenate : Concatenate  NumInputs=3  Mode=Multidimensional array  ConcatenateDimension=2
  Mux1 : Mux  Inputs=3
  Mux2 : Mux  Inputs=3
  Mux3 : Mux  Inputs=3
  Product : Product  Multiplication=Matrix(*)
  I_alfa : Outport  VectorParamsAs1DForOutWhenUnconnected=off
  I_beta : Outport  Port=2  VectorParamsAs1DForOutWhenUnconnected=off
  I_0 : Outport  Port=3  VectorParamsAs1DForOutWhenUnconnected=off
  wires:
  Constant/1 -> Mux1/1
  Constant1/1 -> Mux1/2
  Constant2/1 -> Mux1/3
  Constant3/1 -> Mux2/1
  Constant4/1 -> Mux2/2
  Constant5/1 -> Mux2/3
  Constant6/1 -> Mux3/1
  Constant7/1 -> Mux3/2
  Constant8/1 -> Mux3/3
  Math Function/1 -> Gain/1
  Matrix Concatenate/1 -> Math Function/1
  Mux2/1 -> Matrix Concatenate/2
  Mux3/1 -> Matrix Concatenate/3
  Mux1/1 -> Matrix Concatenate/1
  Product/1 -> Demux/1
  Demux/1 -> I_alfa/1
  Demux/2 -> I_beta/1
  Demux/3 -> I_0/1
  Gain/1 -> Display/1, Product/1
  Isum/1 -> Product/2
